simulink library "mech_flexible_element_lib"  (Simulink 7.1)
PreLoadFcn:
  | oldWarningState = warning('query');
  | warning('off');
PostLoadFcn:
  | find_system(gcs,'FollowLinks', 'on', 'LookUnderMasks', 'all');
  | lastwarn('');
  | warning(oldWarningState);
libraries: mblibv1 x29
settings Model: Creator=arnav  LastModifiedBy=batserve  ExtModeAutoUpdateStatusClock=off

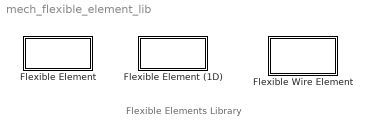
== system mech_flexible_element_lib ==
  note: Flexible Elements Library
  Flexible Element : Subsystem  mask{material=Mild Steel, density=7600, crossArea=1E-4, length=0.15, cgLeng=0.075, beamDir=[1 0 0], Inertia=[120 0 0;0 6400.0 0;0 0 6400.0]*1E-7, youngsM=200E9, shearM=26E9, Ixx=8.3333e-010, Iyy=8.3333e-010, matDamping=0.35}
      mask prompts: material "Beam Material"; density "Material Density (Kg/m^3)"; crossArea "Area of cross-section (m^2)"; length "Length of single element (m)"; cgLeng "Distance of CG along length of beam element (m)"; beamDir "Direction of beam element (X direction will be [1 0 0])"; Inertia "Mass Moment of Inertia of beam element (Kg/m^2)"; youngsM "Youngs Modulus (N/m^2)"; shearM "Shear Modulus (N/m^2)"; Ixx "Area Moment of Inertia along the direction of bending (m^4)"; Iyy "Area Moment of Inertia normal to the direction of bending (m^4)"; matDamping "Material Dampening Coefficient"
      mask init:
      | flexBeamElement.material    = material;
      | flexBeamElement.density     = density;
      | flexBeamElement.crossArea   = crossArea;
      | flexBeamElement.length      = length;
      | flexBeamElement.cgLeng      = cgLeng;
      | flexBeamElement.beamDir     = beamDir;
      | flexBeamElement.Inertia     = Inertia;
      | flexBeamElement.youngsM     = youngsM;
      | flexBeamElement.shearM      = shearM;
      | flexBeamElement.Ixx         = Ixx;
      | flexBeamElement.Iyy         = Iyy;
      | flexBeamElement.matDamping  = matDamping;
      | [flexBeamElement] = mech_flexible_beamelement(flexBeamElement);
  Flexible Element (1D) : Subsystem  AncestorBlock=mech_flexible_element_lib/Flexible Element  mask{material=Mild Steel, density=7600, crossArea=1E-4, length=0.15, cgLeng=0.075, beamDir=[1 0 0], Inertia=[120 0 0;0 6400.0 0;0 0 6400.0]*1E-7, youngsM=200E9, shearM=26E9, Ixx=8.3333e-010, Iyy=8.3333e-010, matDamping=0.35}
      mask prompts: material "Beam Material"; density "Material Density (Kg/m^3)"; crossArea "Area of cross-section (m^2)"; length "Length of single element (m)"; cgLeng "Distance of CG along length of beam element (m)"; beamDir "Direction of beam element (X direction will be [1 0 0])"; Inertia "Mass Moment of Inertia of beam element (Kg/m^2)"; youngsM "Youngs Modulus (N/m^2)"; shearM "Shear Modulus (N/m^2)"; Ixx "Area Moment of Inertia along the direction of bending (m^4)"; Iyy "Area Moment of Inertia normal to the direction of bending (m^4)"; matDamping "Material Dampening Coefficient"
      mask init:
      | flexBeamElement.material    = material;
      | flexBeamElement.density     = density;
      | flexBeamElement.crossArea   = crossArea;
      | flexBeamElement.length      = length;
      | flexBeamElement.cgLeng      = cgLeng;
      | flexBeamElement.beamDir     = beamDir;
      | flexBeamElement.Inertia     = Inertia;
      | flexBeamElement.youngsM     = youngsM;
      | flexBeamElement.shearM      = shearM;
      | flexBeamElement.Ixx         = Ixx;
      | flexBeamElement.Iyy         = Ixx;
      | flexBeamElement.matDamping  = matDamping;
      | [flexBeamElement] = mech_flexible_beamelement(flexBeamElement);
  Flexible Wire Element : Subsystem  AncestorBlock=mech_flexible_element_lib/Flexible Element  mask(Flexible wire element){material=Mild Steel, density=7600, wireDia=1E-6, length=0.1, cgLeng=0.05, beamDir=[1 0 0], Inertia=[0.001 0 0;0 5.0 0;0 0 5.0]*1E-7, youngsM=200E9, matDamping=0.1}
      mask prompts: material "Beam Material"; density "Material Density (Kg/m^3)"; wireDia "Wire diameter (m)"; length "Length of single element (m)"; cgLeng "Distance of CG along length of beam element (m)"; beamDir "Direction of beam element (X direction will be [1 0 0])"; Inertia "Mass Moment of Inertia of beam element (Kg/m^2)"; youngsM "Youngs Modulus (N/m^2)"; matDamping "Material Dampening Coefficient"
      mask help: The flexible wire element has a single body that has two degrees of freedom w.r.t its neighbour. It can rotate (bend) and translate along the wire direction (elongate). The material constants and wire dimensions are used to compute the stiffness and damping on these degrees of freedom.
      mask init:
      | flexBeamElement.material    = material;
      | flexBeamElement.density     = density;
      | flexBeamElement.crossArea   = pi*wireDia^2/4;
      | flexBeamElement.length      = length;
      | flexBeamElement.cgLeng      = cgLeng;
      | flexBeamElement.beamDir     = beamDir;
      | flexBeamElement.Inertia     = Inertia;
      | flexBeamElement.youngsM     = youngsM;
      | flexBeamElement.shearM      = 20E9;
      | flexBeamElement.Ixx         = pi*wireDia^4/64;
      | flexBeamElement.Iyy         = pi*wireDia^4/64;
      | flexBeamElement.matDamping  = matDamping;
      | [flexBeamElement] = mech_flexible_beamelement(flexBeamElement);

== system mech_flexible_element_lib/Flexible Element ==
  FlexibleElement : Subsystem
  Base : PMIOPort  Port=1  Side=Left
  Tip : PMIOPort  Orientation=left  Port=2  Side=Right
  connections:
  FlexibleElement/RConn1 -- Tip/RConn1
  Base/RConn1 -- FlexibleElement/LConn1

== system mech_flexible_element_lib/Flexible Element (1D) ==
  FlexibleElement : Subsystem
  Base : PMIOPort  Port=1  Side=Left
  Tip : PMIOPort  Orientation=left  Port=2  Side=Right
  connections:
  Base/RConn1 -- FlexibleElement/LConn1
  FlexibleElement/RConn1 -- Tip/RConn1

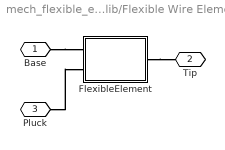
== system mech_flexible_element_lib/Flexible Wire Element ==
  FlexibleElement : Subsystem
  Base : PMIOPort  Port=1  Side=Left
  Tip : PMIOPort  Orientation=left  Port=2  Side=Right
  Pluck : PMIOPort  Port=3  Side=Left
  connections:
  Base/RConn1 -- FlexibleElement/LConn1
  FlexibleElement/RConn1 -- Tip/RConn1
  Pluck/RConn1 -- FlexibleElement/LConn2

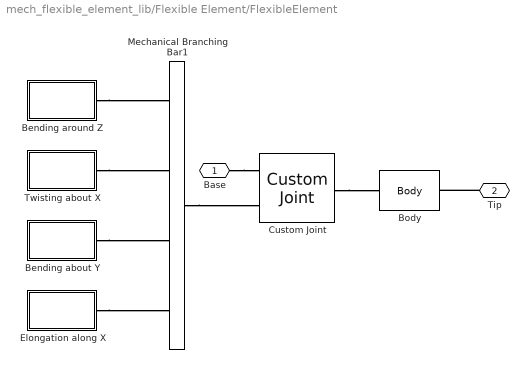
== system mech_flexible_element_lib/Flexible Element/FlexibleElement ==
  Bending about Y : Subsystem  Orientation=left
  Bending around Z : Subsystem  Orientation=left
  Body : mblibv1/Bodies/Body  DialogController=MECH.DynMechDlgSource  PhysicalDomain=mechanical  SubClassName=Unknown  LeftPortType=workingframe  RightPortType=workingframe  LConnTagsString=CS1  RConnTagsString=CS2  DialogClass=MechanicalBodyBlock  Mass=flexBeamElement.mass  MassUnits=kg  InertiaUnits=kg*m^2  Inertia=flexBeamElement.Inertia  Shape=Cylinder  ShapeDims=[1 1]  ShapeUnits=m  ShapeUse=false  Density=1  DensityUnits=kg/m^3  DensityUse=false  GraphicsMode=1  BodyColor=[0.5 0.5 0.5]  GraphicsObj=[]  AttachedToCS=1  CG=Left$CG$flexBeamElement.cg$CS1$CS1$m$[0 0 0]$Euler X-Y-Z$deg$WORLD$false  WorkingFrames=Left$CS1$flexBeamElement.cs1$ADJOINING$ADJOINING$m$[0 0 0]$Euler X-Y-Z$deg$WORLD$true#Right$CS2$flexBeamElement.cs2$CS1$CS1$m$[0 0 0]$Euler X-Y-Z$deg$WORLD$true  CGPos=flexBeamElement.cg  CGRot=[0 0 0]  CS0Pos=[]  CS0Rot=[]  CS1Pos=flexBeamElement.cs1  CS1Rot=[0 0 0]  CS2Pos=flexBeamElement.cs2  CS2Rot=[0 0 0]  CS3Pos=[]  CS3Rot=[]  CS4Pos=[]  CS4Rot=[]  CS5Pos=[]  CS5Rot=[]  CS6Pos=[]  CS6Rot=[]  CS7Pos=[]  CS7Rot=[]  CS8Pos=[]  CS8Rot=[]  CS9Pos=[]  CS9Rot=[]  CS10Pos=[]  CS10Rot=[]  CS11Pos=[]  CS11Rot=[]  CS12Pos=[]  CS12Rot=[]  CS13Pos=[]  CS13Rot=[]  CS14Pos=[]  CS14Rot=[]  CS15Pos=[]  CS15Rot=[]  CS16Pos=[]  CS16Rot=[]  CS17Pos=[]  CS17Rot=[]  CS18Pos=[]  CS18Rot=[]  CS19Pos=[]  CS19Rot=[]  CS20Pos=[]  CS20Rot=[]
  Custom Joint : mblibv1/Joints/Custom Joint  DialogController=MECH.DynMechDlgSource  PhysicalDomain=mechanical  SubClassName=custom_joint  LeftPortType=blob  RightPortType=blob  LConnTagsString=__newl0|SA1  RConnTagsString=__newr0  NumSAPorts=1  CutJoint=off  MarkAsCut=off  Primitives=revolute_revolute_revolute_prismatic  PrimitiveProps=R3$WORLD$flexBeamElement.zDir$revolute#R1$WORLD$flexBeamElement.xDir$revolute#R2$WORLD$flexBeamElement.yDir$revolute#P1$WORLD$flexBeamElement.xDir$prismatic  DialogClass=JointBlock  R1Axis=flexBeamElement.xDir  R2Axis=flexBeamElement.yDir  R3Axis=flexBeamElement.zDir  P1Axis=flexBeamElement.xDir  P2Axis=[]  P3Axis=[]  SAxis=[]
  Elongation along X : Subsystem  Orientation=left
  Mechanical Branching Bar1 : mblibv1/Utilities/Mechanical Branching Bar  Orientation=left  DialogController=MECH.DynMechDlgSource  PhysicalDomain=mechanical  SubClassName=Unknown  LeftPortType=blob  RightPortType=blob  LConnTagsString=_newl0  RConnTagsString=SA0|SA1|SA2|SA3  DialogClass=MechanicalBranchingBarBlock  NumSAPorts=4
  Twisting about X : Subsystem  Orientation=left
  Base : PMIOPort  Port=1  Side=Left
  Tip : PMIOPort  Orientation=left  Port=2  Side=Right
  connections:
  Tip/RConn1 -- Body/RConn1
  Custom Joint/RConn1 -- Body/LConn1
  Base/RConn1 -- Custom Joint/LConn1
  Mechanical Branching Bar1/LConn1 -- Custom Joint/LConn2
  Bending around Z/LConn1 -- Mechanical Branching Bar1/RConn1
  Twisting about X/LConn1 -- Mechanical Branching Bar1/RConn2
  Bending about Y/LConn1 -- Mechanical Branching Bar1/RConn3
  Elongation along X/LConn1 -- Mechanical Branching Bar1/RConn4

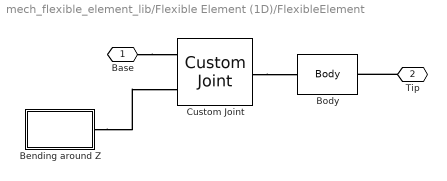
== system mech_flexible_element_lib/Flexible Element (1D)/FlexibleElement ==
  Bending around Z : Subsystem  Orientation=left
  Body : mblibv1/Bodies/Body  DialogController=MECH.DynMechDlgSource  PhysicalDomain=mechanical  SubClassName=Unknown  LeftPortType=workingframe  RightPortType=workingframe  LConnTagsString=CS1  RConnTagsString=CS2  DialogClass=MechanicalBodyBlock  Mass=flexBeamElement.mass  MassUnits=kg  InertiaUnits=kg*m^2  Inertia=flexBeamElement.Inertia  Shape=Cylinder  ShapeDims=[1 1]  ShapeUnits=m  ShapeUse=false  Density=1  DensityUnits=kg/m^3  DensityUse=false  GraphicsMode=1  BodyColor=[0.5 0.5 0.5]  GraphicsObj=[]  AttachedToCS=1  CG=Left$CG$flexBeamElement.cg$CS1$CS1$m$[0 0 0]$Euler X-Y-Z$deg$WORLD$false  WorkingFrames=Left$CS1$flexBeamElement.cs1$ADJOINING$ADJOINING$m$[0 0 0]$Euler X-Y-Z$deg$WORLD$true#Right$CS2$flexBeamElement.cs2$CS1$CS1$m$[0 0 0]$Euler X-Y-Z$deg$WORLD$true  CGPos=flexBeamElement.cg  CGRot=[0 0 0]  CS0Pos=[]  CS0Rot=[]  CS1Pos=flexBeamElement.cs1  CS1Rot=[0 0 0]  CS2Pos=flexBeamElement.cs2  CS2Rot=[0 0 0]  CS3Pos=[]  CS3Rot=[]  CS4Pos=[]  CS4Rot=[]  CS5Pos=[]  CS5Rot=[]  CS6Pos=[]  CS6Rot=[]  CS7Pos=[]  CS7Rot=[]  CS8Pos=[]  CS8Rot=[]  CS9Pos=[]  CS9Rot=[]  CS10Pos=[]  CS10Rot=[]  CS11Pos=[]  CS11Rot=[]  CS12Pos=[]  CS12Rot=[]  CS13Pos=[]  CS13Rot=[]  CS14Pos=[]  CS14Rot=[]  CS15Pos=[]  CS15Rot=[]  CS16Pos=[]  CS16Rot=[]  CS17Pos=[]  CS17Rot=[]  CS18Pos=[]  CS18Rot=[]  CS19Pos=[]  CS19Rot=[]  CS20Pos=[]  CS20Rot=[]
  Custom Joint : mblibv1/Joints/Custom Joint  DialogController=MECH.DynMechDlgSource  PhysicalDomain=mechanical  SubClassName=custom_joint  LeftPortType=blob  RightPortType=blob  LConnTagsString=__newl0|SA1  RConnTagsString=__newr0  NumSAPorts=1  CutJoint=off  MarkAsCut=off  Primitives=revolute  PrimitiveProps=R3$WORLD$flexBeamElement.zDir$revolute  DialogClass=JointBlock  R1Axis=[]  R2Axis=[]  R3Axis=flexBeamElement.zDir  P1Axis=[]  P2Axis=[]  P3Axis=[]  SAxis=[]
  Base : PMIOPort  Port=1  Side=Left
  Tip : PMIOPort  Orientation=left  Port=2  Side=Right
  connections:
  Base/RConn1 -- Custom Joint/LConn1
  Custom Joint/RConn1 -- Body/LConn1
  Tip/RConn1 -- Body/RConn1
  Bending around Z/LConn1 -- Custom Joint/LConn2

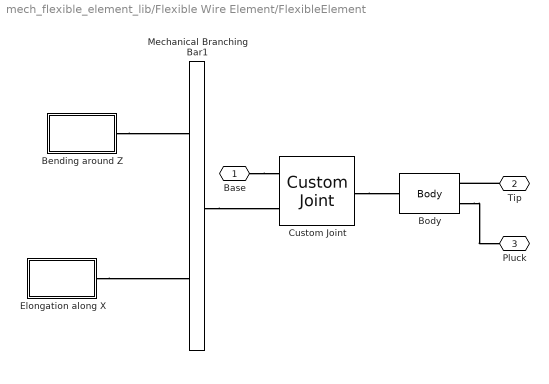
== system mech_flexible_element_lib/Flexible Wire Element/FlexibleElement ==
  Bending around Z : Subsystem  Orientation=left
  Body : mblibv1/Bodies/Body  DialogController=MECH.DynMechDlgSource  PhysicalDomain=mechanical  SubClassName=Unknown  LeftPortType=workingframe  RightPortType=workingframe  LConnTagsString=CS1  RConnTagsString=CS2|CS3  DialogClass=MechanicalBodyBlock  Mass=flexBeamElement.mass  MassUnits=kg  InertiaUnits=kg*m^2  Inertia=flexBeamElement.Inertia  Shape=Cylinder  ShapeDims=[1 1]  ShapeUnits=m  ShapeUse=false  Density=1  DensityUnits=kg/m^3  DensityUse=false  GraphicsMode=1  BodyColor=[0.5 0.5 0.5]  GraphicsObj=[]  AttachedToCS=1  CG=Left$CG$flexBeamElement.cg$CS1$CS1$m$[0 0 0]$Euler X-Y-Z$deg$WORLD$false  WorkingFrames=Left$CS1$flexBeamElement.cs1$ADJOINING$ADJOINING$m$[0 0 0]$Euler X-Y-Z$deg$WORLD$true#Right$CS2$flexBeamElement.cs2$CS1$CS1$m$[0 0 0]$Euler X-Y-Z$deg$WORLD$true#Right$CS3$flexBeamElement.cs2$CS1$CS1$m$[0 0 0]$Euler X-Y-Z$deg$WORLD$true  CGPos=flexBeamElement.cg  CGRot=[0 0 0]  CS0Pos=[]  CS0Rot=[]  CS1Pos=flexBeamElement.cs1  CS1Rot=[0 0 0]  CS2Pos=flexBeamElement.cs2  CS2Rot=[0 0 0]  CS3Pos=flexBeamElement.cs2  CS3Rot=[0 0 0]  CS4Pos=[]  CS4Rot=[]  CS5Pos=[]  CS5Rot=[]  CS6Pos=[]  CS6Rot=[]  CS7Pos=[]  CS7Rot=[]  CS8Pos=[]  CS8Rot=[]  CS9Pos=[]  CS9Rot=[]  CS10Pos=[]  CS10Rot=[]  CS11Pos=[]  CS11Rot=[]  CS12Pos=[]  CS12Rot=[]  CS13Pos=[]  CS13Rot=[]  CS14Pos=[]  CS14Rot=[]  CS15Pos=[]  CS15Rot=[]  CS16Pos=[]  CS16Rot=[]  CS17Pos=[]  CS17Rot=[]  CS18Pos=[]  CS18Rot=[]  CS19Pos=[]  CS19Rot=[]  CS20Pos=[]  CS20Rot=[]
  Custom Joint : mblibv1/Joints/Custom Joint  DialogController=MECH.DynMechDlgSource  PhysicalDomain=mechanical  SubClassName=custom_joint  LeftPortType=blob  RightPortType=blob  LConnTagsString=__newl0|SA1  RConnTagsString=__newr0  NumSAPorts=1  CutJoint=off  MarkAsCut=off  Primitives=revolute_prismatic  PrimitiveProps=R3$WORLD$flexBeamElement.zDir$revolute#P1$WORLD$flexBeamElement.xDir$prismatic  DialogClass=JointBlock  R1Axis=[]  R2Axis=[]  R3Axis=flexBeamElement.zDir  P1Axis=flexBeamElement.xDir  P2Axis=[]  P3Axis=[]  SAxis=[]
  Elongation along X : Subsystem  Orientation=left
  Mechanical Branching Bar1 : mblibv1/Utilities/Mechanical Branching Bar  Orientation=left  DialogController=MECH.DynMechDlgSource  PhysicalDomain=mechanical  SubClassName=Unknown  LeftPortType=blob  RightPortType=blob  LConnTagsString=_newl0  RConnTagsString=SA0|SA1  DialogClass=MechanicalBranchingBarBlock  NumSAPorts=2
  Base : PMIOPort  Port=1  Side=Left
  Tip : PMIOPort  Orientation=left  Port=2  Side=Right
  Pluck : PMIOPort  Orientation=left  Port=3  Side=Left
  connections:
  Elongation along X/LConn1 -- Mechanical Branching Bar1/RConn2
  Bending around Z/LConn1 -- Mechanical Branching Bar1/RConn1
  Mechanical Branching Bar1/LConn1 -- Custom Joint/LConn2
  Base/RConn1 -- Custom Joint/LConn1
  Custom Joint/RConn1 -- Body/LConn1
  Tip/RConn1 -- Body/RConn1
  Body/RConn2 -- Pluck/RConn1

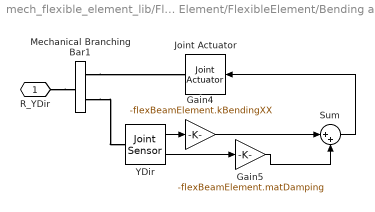
== system mech_flexible_element_lib/Flexible Element/FlexibleElement/Bending about Y ==
  Gain4 : Gain  Gain=-flexBeamElement.kBendingXX  ParameterDataType=sfix(16)  ParameterScaling=2^0  OutDataType=sfix(16)  OutScaling=2^0
  Gain5 : Gain  Gain=-flexBeamElement.matDamping  ParameterDataType=sfix(16)  ParameterScaling=2^0  OutDataType=sfix(16)  OutScaling=2^0
  Joint Actuator : mblibv1/Sensors &  Actuators/Joint Actuator  Orientation=left  DialogController=MECH.DynMechDlgSource  SystemSampleTime=-1  PhysicalDomain=Mechanical  PortType=blob  ActuationStyle=Force  AngleUnits=deg  ArcVelocityUnits=deg/s  ArcAccelerationUnits=deg/s^2  CoordPositionUnits=m  VelocityUnits=m/s  AccelerationUnits=m/s^2  ForceUnits=N  TorqueUnits=N-m  ActiveIO=off  Width=1  DialogClass=MechanicalActuatorBlock  Primitive=R2  ReferenceFrame=Absolute (INERTIAL)
  Mechanical Branching Bar1 : mblibv1/Utilities/Mechanical Branching Bar  DialogController=MECH.DynMechDlgSource  PhysicalDomain=mechanical  SubClassName=Unknown  LeftPortType=blob  RightPortType=blob  LConnTagsString=_newl0  RConnTagsString=SA0|SA1  DialogClass=MechanicalBranchingBarBlock  NumSAPorts=2
  Sum : Sum  Inputs=|++  OutDataType=sfix(16)  OutScaling=2^0
  YDir : mblibv1/Sensors &  Actuators/Joint Sensor  DialogController=MECH.DynMechDlgSource  SystemSampleTime=-1  PhysicalDomain=Mechanical  PortType=blob  Muxed=off  Pose=off  Angle=on  AngleUnits=rad  ArcVelocity=on  ArcVelocityUnits=rad/s  ArcAcceleration=off  ArcAccelerationUnits=deg/s^2  CoordPosition=on  CoordPositionUnits=m  Velocity=off  VelocityUnits=m/s  Acceleration=off  AccelerationUnits=m/s^2  Quaternion=on  QuaternionDT=off  QuaternionDDT=off  QuaternionUnits=off  OutputVector=[ 1 1 ]  ActiveIO=off  Width=2  DialogClass=MechanicalSensorBlock  Primitive=R2  Force=off  ForceUnits=N  Torque=off  TorqueUnits=N-m  ReferenceFrame=Absolute (INERTIAL)  ReactionSensedSide=Base  ReactionReferenceFrame=Absolute (World)  ReactionForce=off  ReactionForceUnits=N  ReactionMoment=off  ReactionMomentUnits=N-m
  R_YDir : PMIOPort  Port=1  Side=Left
  wires:
  YDir/1 -> Gain4/1
  YDir/2 -> Gain5/1
  Gain4/1 -> Sum/1
  Gain5/1 -> Sum/2
  Sum/1 -> Joint Actuator/1
  connections:
  Mechanical Branching Bar1/RConn1 -- Joint Actuator/RConn1
  R_YDir/RConn1 -- Mechanical Branching Bar1/LConn1
  Mechanical Branching Bar1/RConn2 -- YDir/LConn1

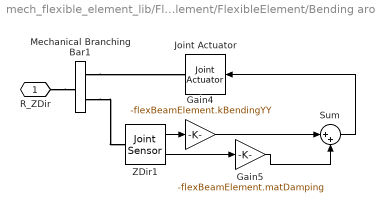
== system mech_flexible_element_lib/Flexible Element/FlexibleElement/Bending around Z ==
  Gain4 : Gain  Gain=-flexBeamElement.kBendingYY  ParameterDataType=sfix(16)  ParameterScaling=2^0  OutDataType=sfix(16)  OutScaling=2^0
  Gain5 : Gain  Gain=-flexBeamElement.matDamping  ParameterDataType=sfix(16)  ParameterScaling=2^0  OutDataType=sfix(16)  OutScaling=2^0
  Joint Actuator : mblibv1/Sensors &  Actuators/Joint Actuator  Orientation=left  DialogController=MECH.DynMechDlgSource  SystemSampleTime=-1  PhysicalDomain=Mechanical  PortType=blob  ActuationStyle=Force  AngleUnits=deg  ArcVelocityUnits=deg/s  ArcAccelerationUnits=deg/s^2  CoordPositionUnits=m  VelocityUnits=m/s  AccelerationUnits=m/s^2  ForceUnits=N  TorqueUnits=N-m  ActiveIO=off  Width=1  DialogClass=MechanicalActuatorBlock  Primitive=R3  ReferenceFrame=Absolute (INERTIAL)
  Mechanical Branching Bar1 : mblibv1/Utilities/Mechanical Branching Bar  DialogController=MECH.DynMechDlgSource  PhysicalDomain=mechanical  SubClassName=Unknown  LeftPortType=blob  RightPortType=blob  LConnTagsString=_newl0  RConnTagsString=SA0|SA1  DialogClass=MechanicalBranchingBarBlock  NumSAPorts=2
  Sum : Sum  Inputs=|++  OutDataType=sfix(16)  OutScaling=2^0
  ZDir1 : mblibv1/Sensors &  Actuators/Joint Sensor  DialogController=MECH.DynMechDlgSource  SystemSampleTime=-1  PhysicalDomain=Mechanical  PortType=blob  Muxed=off  Pose=off  Angle=on  AngleUnits=rad  ArcVelocity=on  ArcVelocityUnits=rad/s  ArcAcceleration=off  ArcAccelerationUnits=deg/s^2  CoordPosition=on  CoordPositionUnits=m  Velocity=off  VelocityUnits=m/s  Acceleration=off  AccelerationUnits=m/s^2  Quaternion=on  QuaternionDT=off  QuaternionDDT=off  QuaternionUnits=off  OutputVector=[ 1 1 ]  ActiveIO=off  Width=2  DialogClass=MechanicalSensorBlock  Primitive=R3  Force=off  ForceUnits=N  Torque=off  TorqueUnits=N-m  ReferenceFrame=Absolute (INERTIAL)  ReactionSensedSide=Base  ReactionReferenceFrame=Absolute (World)  ReactionForce=off  ReactionForceUnits=N  ReactionMoment=off  ReactionMomentUnits=N-m
  R_ZDir : PMIOPort  Port=1  Side=Left
  wires:
  ZDir1/1 -> Gain4/1
  ZDir1/2 -> Gain5/1
  Gain4/1 -> Sum/1
  Gain5/1 -> Sum/2
  Sum/1 -> Joint Actuator/1
  connections:
  Mechanical Branching Bar1/RConn1 -- Joint Actuator/RConn1
  R_ZDir/RConn1 -- Mechanical Branching Bar1/LConn1
  Mechanical Branching Bar1/RConn2 -- ZDir1/LConn1

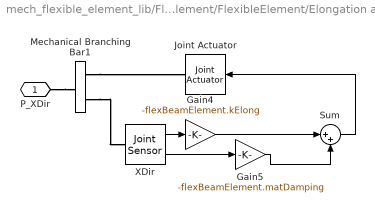
== system mech_flexible_element_lib/Flexible Element/FlexibleElement/Elongation along X ==
  Gain4 : Gain  Gain=-flexBeamElement.kElong  ParameterDataType=sfix(16)  ParameterScaling=2^0  OutDataType=sfix(16)  OutScaling=2^0
  Gain5 : Gain  Gain=-flexBeamElement.matDamping  ParameterDataType=sfix(16)  ParameterScaling=2^0  OutDataType=sfix(16)  OutScaling=2^0
  Joint Actuator : mblibv1/Sensors &  Actuators/Joint Actuator  Orientation=left  DialogController=MECH.DynMechDlgSource  SystemSampleTime=-1  PhysicalDomain=Mechanical  PortType=blob  ActuationStyle=Force  AngleUnits=deg  ArcVelocityUnits=deg/s  ArcAccelerationUnits=deg/s^2  CoordPositionUnits=m  VelocityUnits=m/s  AccelerationUnits=m/s^2  ForceUnits=N  TorqueUnits=N-m  ActiveIO=off  Width=1  DialogClass=MechanicalActuatorBlock  Primitive=P1  ReferenceFrame=Absolute (INERTIAL)
  Mechanical Branching Bar1 : mblibv1/Utilities/Mechanical Branching Bar  DialogController=MECH.DynMechDlgSource  PhysicalDomain=mechanical  SubClassName=Unknown  LeftPortType=blob  RightPortType=blob  LConnTagsString=_newl0  RConnTagsString=SA0|SA1  DialogClass=MechanicalBranchingBarBlock  NumSAPorts=2
  Sum : Sum  Inputs=|++  OutDataType=sfix(16)  OutScaling=2^0
  XDir : mblibv1/Sensors &  Actuators/Joint Sensor  DialogController=MECH.DynMechDlgSource  SystemSampleTime=-1  PhysicalDomain=Mechanical  PortType=blob  Muxed=off  Pose=off  Angle=on  AngleUnits=rad  ArcVelocity=on  ArcVelocityUnits=rad/s  ArcAcceleration=off  ArcAccelerationUnits=deg/s^2  CoordPosition=on  CoordPositionUnits=m  Velocity=on  VelocityUnits=m/s  Acceleration=off  AccelerationUnits=m/s^2  Quaternion=on  QuaternionDT=off  QuaternionDDT=off  QuaternionUnits=off  OutputVector=[ 1 1 ]  ActiveIO=off  Width=2  DialogClass=MechanicalSensorBlock  Primitive=P1  Force=off  ForceUnits=N  Torque=off  TorqueUnits=N-m  ReferenceFrame=Absolute (INERTIAL)  ReactionSensedSide=Base  ReactionReferenceFrame=Absolute (World)  ReactionForce=off  ReactionForceUnits=N  ReactionMoment=off  ReactionMomentUnits=N-m
  P_XDir : PMIOPort  Port=1  Side=Left
  wires:
  Sum/1 -> Joint Actuator/1
  Gain5/1 -> Sum/2
  Gain4/1 -> Sum/1
  XDir/2 -> Gain5/1
  XDir/1 -> Gain4/1
  connections:
  Mechanical Branching Bar1/RConn2 -- XDir/LConn1
  P_XDir/RConn1 -- Mechanical Branching Bar1/LConn1
  Mechanical Branching Bar1/RConn1 -- Joint Actuator/RConn1

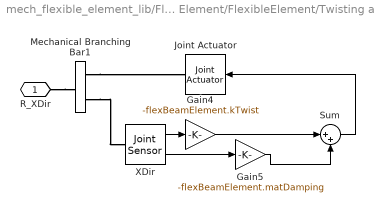
== system mech_flexible_element_lib/Flexible Element/FlexibleElement/Twisting about X ==
  Gain4 : Gain  Gain=-flexBeamElement.kTwist  ParameterDataType=sfix(16)  ParameterScaling=2^0  OutDataType=sfix(16)  OutScaling=2^0
  Gain5 : Gain  Gain=-flexBeamElement.matDamping  ParameterDataType=sfix(16)  ParameterScaling=2^0  OutDataType=sfix(16)  OutScaling=2^0
  Joint Actuator : mblibv1/Sensors &  Actuators/Joint Actuator  Orientation=left  DialogController=MECH.DynMechDlgSource  SystemSampleTime=-1  PhysicalDomain=Mechanical  PortType=blob  ActuationStyle=Force  AngleUnits=deg  ArcVelocityUnits=deg/s  ArcAccelerationUnits=deg/s^2  CoordPositionUnits=m  VelocityUnits=m/s  AccelerationUnits=m/s^2  ForceUnits=N  TorqueUnits=N-m  ActiveIO=off  Width=1  DialogClass=MechanicalActuatorBlock  Primitive=R1  ReferenceFrame=Absolute (INERTIAL)
  Mechanical Branching Bar1 : mblibv1/Utilities/Mechanical Branching Bar  DialogController=MECH.DynMechDlgSource  PhysicalDomain=mechanical  SubClassName=Unknown  LeftPortType=blob  RightPortType=blob  LConnTagsString=_newl0  RConnTagsString=SA0|SA1  DialogClass=MechanicalBranchingBarBlock  NumSAPorts=2
  Sum : Sum  Inputs=|++  OutDataType=sfix(16)  OutScaling=2^0
  XDir : mblibv1/Sensors &  Actuators/Joint Sensor  DialogController=MECH.DynMechDlgSource  SystemSampleTime=-1  PhysicalDomain=Mechanical  PortType=blob  Muxed=off  Pose=off  Angle=on  AngleUnits=rad  ArcVelocity=on  ArcVelocityUnits=rad/s  ArcAcceleration=off  ArcAccelerationUnits=deg/s^2  CoordPosition=on  CoordPositionUnits=m  Velocity=off  VelocityUnits=m/s  Acceleration=off  AccelerationUnits=m/s^2  Quaternion=on  QuaternionDT=off  QuaternionDDT=off  QuaternionUnits=off  OutputVector=[ 1 1 ]  ActiveIO=off  Width=2  DialogClass=MechanicalSensorBlock  Primitive=R1  Force=off  ForceUnits=N  Torque=off  TorqueUnits=N-m  ReferenceFrame=Absolute (INERTIAL)  ReactionSensedSide=Base  ReactionReferenceFrame=Absolute (World)  ReactionForce=off  ReactionForceUnits=N  ReactionMoment=off  ReactionMomentUnits=N-m
  R_XDir : PMIOPort  Port=1  Side=Left
  wires:
  Sum/1 -> Joint Actuator/1
  Gain5/1 -> Sum/2
  Gain4/1 -> Sum/1
  XDir/2 -> Gain5/1
  XDir/1 -> Gain4/1
  connections:
  Mechanical Branching Bar1/RConn2 -- XDir/LConn1
  R_XDir/RConn1 -- Mechanical Branching Bar1/LConn1
  Mechanical Branching Bar1/RConn1 -- Joint Actuator/RConn1

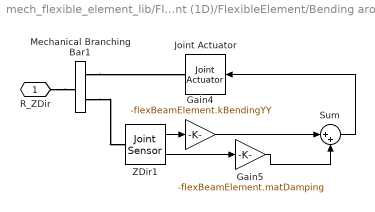
== system mech_flexible_element_lib/Flexible Element (1D)/FlexibleElement/Bending around Z ==
  Gain4 : Gain  Gain=-flexBeamElement.kBendingYY  ParameterDataType=sfix(16)  ParameterScaling=2^0  OutDataType=sfix(16)  OutScaling=2^0
  Gain5 : Gain  Gain=-flexBeamElement.matDamping  ParameterDataType=sfix(16)  ParameterScaling=2^0  OutDataType=sfix(16)  OutScaling=2^0
  Joint Actuator : mblibv1/Sensors &  Actuators/Joint Actuator  Orientation=left  DialogController=MECH.DynMechDlgSource  SystemSampleTime=-1  PhysicalDomain=Mechanical  PortType=blob  ActuationStyle=Force  AngleUnits=deg  ArcVelocityUnits=deg/s  ArcAccelerationUnits=deg/s^2  CoordPositionUnits=m  VelocityUnits=m/s  AccelerationUnits=m/s^2  ForceUnits=N  TorqueUnits=N-m  ActiveIO=off  Width=1  DialogClass=MechanicalActuatorBlock  Primitive=R3  ReferenceFrame=Absolute (INERTIAL)
  Mechanical Branching Bar1 : mblibv1/Utilities/Mechanical Branching Bar  DialogController=MECH.DynMechDlgSource  PhysicalDomain=mechanical  SubClassName=Unknown  LeftPortType=blob  RightPortType=blob  LConnTagsString=_newl0  RConnTagsString=SA0|SA1  DialogClass=MechanicalBranchingBarBlock  NumSAPorts=2
  Sum : Sum  Inputs=|++  OutDataType=sfix(16)  OutScaling=2^0
  ZDir1 : mblibv1/Sensors &  Actuators/Joint Sensor  DialogController=MECH.DynMechDlgSource  SystemSampleTime=-1  PhysicalDomain=Mechanical  PortType=blob  Muxed=off  Pose=off  Angle=on  AngleUnits=rad  ArcVelocity=on  ArcVelocityUnits=rad/s  ArcAcceleration=off  ArcAccelerationUnits=deg/s^2  CoordPosition=on  CoordPositionUnits=m  Velocity=off  VelocityUnits=m/s  Acceleration=off  AccelerationUnits=m/s^2  Quaternion=on  QuaternionDT=off  QuaternionDDT=off  QuaternionUnits=off  OutputVector=[ 1 1 ]  ActiveIO=off  Width=2  DialogClass=MechanicalSensorBlock  Primitive=R3  Force=off  ForceUnits=N  Torque=off  TorqueUnits=N-m  ReferenceFrame=Absolute (INERTIAL)  ReactionSensedSide=Base  ReactionReferenceFrame=Absolute (World)  ReactionForce=off  ReactionForceUnits=N  ReactionMoment=off  ReactionMomentUnits=N-m
  R_ZDir : PMIOPort  Port=1  Side=Left
  wires:
  Sum/1 -> Joint Actuator/1
  Gain5/1 -> Sum/2
  Gain4/1 -> Sum/1
  ZDir1/2 -> Gain5/1
  ZDir1/1 -> Gain4/1
  connections:
  Mechanical Branching Bar1/RConn2 -- ZDir1/LConn1
  R_ZDir/RConn1 -- Mechanical Branching Bar1/LConn1
  Mechanical Branching Bar1/RConn1 -- Joint Actuator/RConn1

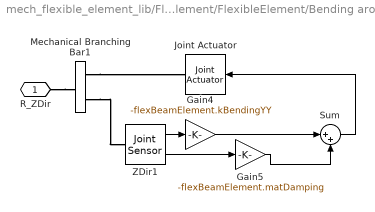
== system mech_flexible_element_lib/Flexible Wire Element/FlexibleElement/Bending around Z ==
  Gain4 : Gain  Gain=-flexBeamElement.kBendingYY  ParameterDataType=sfix(16)  ParameterScaling=2^0  OutDataType=sfix(16)  OutScaling=2^0
  Gain5 : Gain  Gain=-flexBeamElement.matDamping  ParameterDataType=sfix(16)  ParameterScaling=2^0  OutDataType=sfix(16)  OutScaling=2^0
  Joint Actuator : mblibv1/Sensors &  Actuators/Joint Actuator  Orientation=left  DialogController=MECH.DynMechDlgSource  SystemSampleTime=-1  PhysicalDomain=Mechanical  PortType=blob  ActuationStyle=Force  AngleUnits=deg  ArcVelocityUnits=deg/s  ArcAccelerationUnits=deg/s^2  CoordPositionUnits=m  VelocityUnits=m/s  AccelerationUnits=m/s^2  ForceUnits=N  TorqueUnits=N-m  ActiveIO=off  Width=1  DialogClass=MechanicalActuatorBlock  Primitive=R3  ReferenceFrame=Absolute (INERTIAL)
  Mechanical Branching Bar1 : mblibv1/Utilities/Mechanical Branching Bar  DialogController=MECH.DynMechDlgSource  PhysicalDomain=mechanical  SubClassName=Unknown  LeftPortType=blob  RightPortType=blob  LConnTagsString=_newl0  RConnTagsString=SA0|SA1  DialogClass=MechanicalBranchingBarBlock  NumSAPorts=2
  Sum : Sum  Inputs=|++  OutDataType=sfix(16)  OutScaling=2^0
  ZDir1 : mblibv1/Sensors &  Actuators/Joint Sensor  DialogController=MECH.DynMechDlgSource  SystemSampleTime=-1  PhysicalDomain=Mechanical  PortType=blob  Muxed=off  Pose=off  Angle=on  AngleUnits=rad  ArcVelocity=on  ArcVelocityUnits=rad/s  ArcAcceleration=off  ArcAccelerationUnits=deg/s^2  CoordPosition=on  CoordPositionUnits=m  Velocity=off  VelocityUnits=m/s  Acceleration=off  AccelerationUnits=m/s^2  Quaternion=on  QuaternionDT=off  QuaternionDDT=off  QuaternionUnits=off  OutputVector=[ 1 1 ]  ActiveIO=off  Width=2  DialogClass=MechanicalSensorBlock  Primitive=R3  Force=off  ForceUnits=N  Torque=off  TorqueUnits=N-m  ReferenceFrame=Absolute (INERTIAL)  ReactionSensedSide=Base  ReactionReferenceFrame=Absolute (World)  ReactionForce=off  ReactionForceUnits=N  ReactionMoment=off  ReactionMomentUnits=N-m
  R_ZDir : PMIOPort  Port=1  Side=Left
  wires:
  Sum/1 -> Joint Actuator/1
  Gain5/1 -> Sum/2
  Gain4/1 -> Sum/1
  ZDir1/2 -> Gain5/1
  ZDir1/1 -> Gain4/1
  connections:
  Mechanical Branching Bar1/RConn2 -- ZDir1/LConn1
  R_ZDir/RConn1 -- Mechanical Branching Bar1/LConn1
  Mechanical Branching Bar1/RConn1 -- Joint Actuator/RConn1

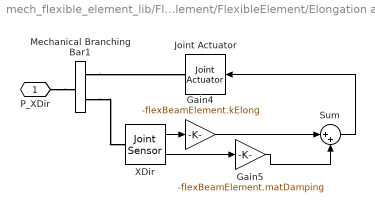
== system mech_flexible_element_lib/Flexible Wire Element/FlexibleElement/Elongation along X ==
  Gain4 : Gain  Gain=-flexBeamElement.kElong  ParameterDataType=sfix(16)  ParameterScaling=2^0  OutDataType=sfix(16)  OutScaling=2^0
  Gain5 : Gain  Gain=-flexBeamElement.matDamping  ParameterDataType=sfix(16)  ParameterScaling=2^0  OutDataType=sfix(16)  OutScaling=2^0
  Joint Actuator : mblibv1/Sensors &  Actuators/Joint Actuator  Orientation=left  DialogController=MECH.DynMechDlgSource  SystemSampleTime=-1  PhysicalDomain=Mechanical  PortType=blob  ActuationStyle=Force  AngleUnits=deg  ArcVelocityUnits=deg/s  ArcAccelerationUnits=deg/s^2  CoordPositionUnits=m  VelocityUnits=m/s  AccelerationUnits=m/s^2  ForceUnits=N  TorqueUnits=N-m  ActiveIO=off  Width=1  DialogClass=MechanicalActuatorBlock  Primitive=P1  ReferenceFrame=Absolute (INERTIAL)
  Mechanical Branching Bar1 : mblibv1/Utilities/Mechanical Branching Bar  DialogController=MECH.DynMechDlgSource  PhysicalDomain=mechanical  SubClassName=Unknown  LeftPortType=blob  RightPortType=blob  LConnTagsString=_newl0  RConnTagsString=SA0|SA1  DialogClass=MechanicalBranchingBarBlock  NumSAPorts=2
  Sum : Sum  Inputs=|++  OutDataType=sfix(16)  OutScaling=2^0
  XDir : mblibv1/Sensors &  Actuators/Joint Sensor  DialogController=MECH.DynMechDlgSource  SystemSampleTime=-1  PhysicalDomain=Mechanical  PortType=blob  Muxed=off  Pose=off  Angle=on  AngleUnits=rad  ArcVelocity=on  ArcVelocityUnits=rad/s  ArcAcceleration=off  ArcAccelerationUnits=deg/s^2  CoordPosition=on  CoordPositionUnits=m  Velocity=on  VelocityUnits=m/s  Acceleration=off  AccelerationUnits=m/s^2  Quaternion=on  QuaternionDT=off  QuaternionDDT=off  QuaternionUnits=off  OutputVector=[ 1 1 ]  ActiveIO=off  Width=2  DialogClass=MechanicalSensorBlock  Primitive=P1  Force=off  ForceUnits=N  Torque=off  TorqueUnits=N-m  ReferenceFrame=Absolute (INERTIAL)  ReactionSensedSide=Base  ReactionReferenceFrame=Absolute (World)  ReactionForce=off  ReactionForceUnits=N  ReactionMoment=off  ReactionMomentUnits=N-m
  P_XDir : PMIOPort  Port=1  Side=Left
  wires:
  XDir/1 -> Gain4/1
  XDir/2 -> Gain5/1
  Gain4/1 -> Sum/1
  Gain5/1 -> Sum/2
  Sum/1 -> Joint Actuator/1
  connections:
  Mechanical Branching Bar1/RConn1 -- Joint Actuator/RConn1
  P_XDir/RConn1 -- Mechanical Branching Bar1/LConn1
  Mechanical Branching Bar1/RConn2 -- XDir/LConn1
